simulink model "RoboticFish_NGC"  (R2023b)
settings: Solver=ode4  StartTime=0.0  StopTime=89  FixedStep=0.00025  RelTol=1e-3  EnableMultiTasking=on
undefined symbols (not defined in the file): Ref, uCMD
libraries: sharedutil x11, slpidlib x8, dspsigops x2, matrix_library x1, SignalEditorBlockLib x1, vrlib x1
(part 3 of 3)

== system RoboticFish_NGC/VRML /Estimate States/Subsystem ==
  Position : Inport
  nu_B : Inport  Port=2
  Bus Creator : BusCreator  Inputs=6
  Bus Creator1 : BusCreator  Inputs=6
  Bus Creator2 : BusCreator  Inputs=2
  Selector : Selector  InputPortWidth=6  IndexOptions=Index vector (dialog)  Indices=[1]  OutputSizes=1
  Selector1 : Selector  InputPortWidth=6  IndexOptions=Index vector (dialog)  Indices=[2]  OutputSizes=1
  Selector10 : Selector  InputPortWidth=6  IndexOptions=Index vector (dialog)  Indices=[5]  OutputSizes=1
  Selector11 : Selector  InputPortWidth=6  IndexOptions=Index vector (dialog)  Indices=[6]  OutputSizes=1
  Selector2 : Selector  InputPortWidth=6  IndexOptions=Index vector (dialog)  Indices=[3]  OutputSizes=1
  Selector3 : Selector  InputPortWidth=6  IndexOptions=Index vector (dialog)  Indices=[4]  OutputSizes=1
  Selector4 : Selector  InputPortWidth=6  IndexOptions=Index vector (dialog)  Indices=[5]  OutputSizes=1
  Selector5 : Selector  InputPortWidth=6  IndexOptions=Index vector (dialog)  Indices=[6]  OutputSizes=1
  Selector6 : Selector  InputPortWidth=6  IndexOptions=Index vector (dialog)  Indices=[1]  OutputSizes=1
  Selector7 : Selector  InputPortWidth=6  IndexOptions=Index vector (dialog)  Indices=[2]  OutputSizes=1
  Selector8 : Selector  InputPortWidth=6  IndexOptions=Index vector (dialog)  Indices=[3]  OutputSizes=1
  Selector9 : Selector  InputPortWidth=6  IndexOptions=Index vector (dialog)  Indices=[4]  OutputSizes=1
  State Estimate : Outport  VectorParamsAs1DForOutWhenUnconnected=off
  wires:
  Position/1 -> Selector5/1, Selector4/1, Selector3/1, Selector2/1, Selector1/1, Selector/1
  Selector/1 -> Bus Creator/1  "X"
  Selector1/1 -> Bus Creator/2  "Y"
  Selector2/1 -> Bus Creator/3  "Z"
  Selector3/1 -> Bus Creator/4  "Roll"
  Selector4/1 -> Bus Creator/5  "Pitch"
  Selector5/1 -> Bus Creator/6  "Yaw"
  nu_B/1 -> Selector8/1, Selector7/1, Selector6/1, Selector11/1, Selector10/1, Selector9/1
  Selector6/1 -> Bus Creator1/1  "u"
  Selector7/1 -> Bus Creator1/2  "v"
  Selector8/1 -> Bus Creator1/3  "w"
  Selector9/1 -> Bus Creator1/4  "p"
  Selector10/1 -> Bus Creator1/5  "q"
  Selector11/1 -> Bus Creator1/6  "r"
  Bus Creator/1 -> Bus Creator2/1  "Position"
  Bus Creator1/1 -> Bus Creator2/2  "Velocity"
  Bus Creator2/1 -> State Estimate/1

== system RoboticFish_NGC/VRML /RF Position and Rotation to VR Translation and Rotation/Orientation to VR Rotation ==
  Orientation : Inport
  Add : Sum  Inputs=4
  Constant1 : Constant  Value=[0; 0; 0; 0]
  Demux : Demux
  Demux1 : Demux
  Gain : Gain  Gain=2
  Gain1 : Gain  Gain=-1
  Gain2 : Gain  Gain=-1
  Math Function : Math  Operator=square  SignedPower=on
  Math Function1 : Math  Operator=reciprocal  SignedPower=on
  Mux : Mux
  Product1 : Product
  Sqrt : Sqrt
  Switch : Switch  Criteria=u2 > Threshold  SaturateOnIntegerOverflow=off  InputSameDT=off
  Trigonometric Function : Trigonometry  Operator=acos
  VR Rotation : Outport  VectorParamsAs1DForOutWhenUnconnected=off
  wires:
  Add/1 -> Sqrt/1
  Demux/2 -> Add/2
  Constant1/1 -> Switch/3
  Demux/3 -> Add/3
  Orientation/1 -> Product1/1, Math Function/1
  Sqrt/1 -> Math Function1/1, Switch/2
  Math Function1/1 -> Product1/2
  Demux/4 -> Add/4
  Demux/1 -> Add/1
  Math Function/1 -> Demux/1
  Product1/1 -> Switch/1
  Trigonometric Function/1 -> Gain/1
  Gain/1 -> Mux/4
  Mux/1 -> VR Rotation/1
  Switch/1 -> Demux1/1
  Demux1/1 -> Trigonometric Function/1  "q0"
  Demux1/2 -> Gain1/1  "q1"
  Demux1/3 -> Mux/1  "q2"
  Demux1/4 -> Gain2/1  "q3"
  Gain2/1 -> Mux/2
  Gain1/1 -> Mux/3

== system RoboticFish_NGC/VRML /RF Position and Rotation to VR Translation and Rotation/Position to VR Translation ==
  Position : Inport
  Demux : Demux  Outputs=3
  Gain : Gain  Gain=-1
  Gain1 : Gain  Gain=-1
  Mux : Mux  Inputs=3
  VR Translation : Outport  VectorParamsAs1DForOutWhenUnconnected=off
  wires:
  Position/1 -> Demux/1
  Demux/1 -> Gain/1  "x"
  Demux/2 -> Mux/1  "y"
  Demux/3 -> Gain1/1  "z"
  Mux/1 -> VR Translation/1
  Gain1/1 -> Mux/2
  Gain/1 -> Mux/3

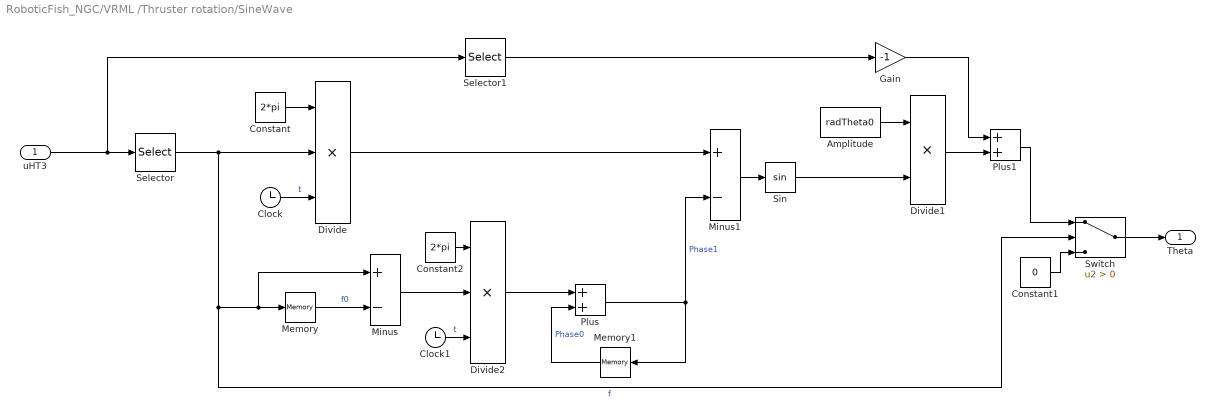
== system RoboticFish_NGC/VRML /Thruster rotation/SineWave ==
  uHT3 : Inport
  Amplitude : Constant  Value=radTheta0
  Clock : Clock
  Clock1 : Clock
  Constant : Constant  Value=2*pi
  Constant1 : Constant  Value=0
  Constant2 : Constant  Value=2*pi
  Divide : Product  Inputs=***
  Divide1 : Product  Inputs=**
  Divide2 : Product  Inputs=***
  Gain : Gain  Gain=-1
  Memory : Memory
  Memory1 : Memory
  Minus : Sum  Inputs=+-
  Minus1 : Sum  Inputs=+-
  Plus : Sum
  Plus1 : Sum
  Selector : Selector  InputPortWidth=2  IndexOptions=Index vector (dialog)  Indices=[1]  OutputSizes=1
  Selector1 : Selector  InputPortWidth=2  IndexOptions=Index vector (dialog)  Indices=[2]  OutputSizes=1
  Sin : Trigonometry
  Switch : Switch  Criteria=u2 > Threshold  SaturateOnIntegerOverflow=off  InputSameDT=off
  Theta : Outport  VectorParamsAs1DForOutWhenUnconnected=off
  wires:
  Constant/1 -> Divide/1
  uHT3/1 -> Selector1/1, Selector/1
  Clock/1 -> Divide/3  "t"
  Amplitude/1 -> Divide1/1
  Memory/1 -> Minus/2  "f0"
  Memory1/1 -> Plus/2  "Phase0"
  Plus/1 -> Memory1/1, Minus1/2  "Phase1"
  Divide/1 -> Minus1/1
  Minus/1 -> Divide2/2
  Divide2/1 -> Plus/1
  Minus1/1 -> Sin/1
  Sin/1 -> Divide1/2
  Selector/1 -> Switch/2, Minus/1, Memory/1, Divide/2  "f"
  Divide1/1 -> Plus1/2
  Selector1/1 -> Gain/1
  Plus1/1 -> Switch/1
  Gain/1 -> Plus1/1
  Constant1/1 -> Switch/3
  Switch/1 -> Theta/1
  Clock1/1 -> Divide2/3  "t"
  Constant2/1 -> Divide2/1

== system RoboticFish_NGC/VRML /WayPoint Position and Rotation To VR Translation and Rotation/Way point Position to VR Translation ==
  Position : Inport
  Demux : Demux  Outputs=3
  Gain : Gain  Gain=-1
  Gain1 : Gain  Gain=-1
  Mux : Mux  Inputs=3
  VR Translation : Outport  VectorParamsAs1DForOutWhenUnconnected=off
  wires:
  Gain/1 -> Mux/3
  Gain1/1 -> Mux/2
  Mux/1 -> VR Translation/1
  Demux/3 -> Gain1/1  "z"
  Demux/2 -> Mux/1  "y"
  Demux/1 -> Gain/1  "x"
  Position/1 -> Demux/1

== system RoboticFish_NGC/Guidance and Control system/ Control system/Control Allocator/Pseudoinverse choice ==
  note: Control Allocation choice
      |
      | The different matrix are used to select different actuators
      | The matrix is T which is the force coefficients pseudoinverse
      | matrix.
      | Matrix 1 - Only lateral propeller for horizontal plane
      | & pectoral fin for depth
      | Matrix 2 - surge motion by means of the caudal fin (HT3) & the
      | lateral propellers for steering & the pectoral fins are used
      | for the depth
      | Matrix 3 -surge force control, 𝜏𝑋, is null. All propellers are
      | switched off.
      | it could happen that the 𝑧 coordinate of the reference has not yet
      | been reached, in which case the control system automatically
      | activates the vertical propeller (VT1) to reach the target
      | Matrix 4 -> utilizza propulsori laterali
      | 𝑇4 + is used both in the case of “Only Propellers” and in the case of “Normal”. In this way the lateral propellers are used as brake. Note that the surge motion control and depth control are treated separately, therefore the force coefficient for the vertical propeller VT1 remains unchanged
      | Matrix 5 -> Only caudal fin
      | Si ha solo la spinta della coda per 𝜏𝑋, non viene compensato nè 𝜏N nè 𝜏Z. Per frenare verrà tolta alimentazione motore e si arriverà al punto desiderato per inerzia.
  Tin : Inport
  Actuators Choice : Inport  Port=2
  Matrix 1 : Constant  Value="[ 0 0 0 ;  0 0 0 ; 0.1 1  0;  0.1 -1  0;  0 0 1 ; 0 0 1  ;0  0 0]"
  Matrix 2 : Constant  Value="[ 1 0 0 ; 0 0 0 ;0 1 0 ;  0 -1 0 ;  0 0 1 ;  0 0 1 ; 0 0 0 ]"
  Matrix 3 : Constant  Value="[ 0 0 0 ;0  0 0; 0 0 0;  0 0 0;  0 0 0; 0 0 0;0 0 1]"
  Matrix 4 : Constant  Value="[ 0 0 0;0 0 0 ; -1 0 0 ;  -1 0 0 ;  0 0  0; 0 0 0;0 0 1]"
  Matrix 5 : Constant  Value="[ 1 0 0; 0 1 0; 0 0 0;  0 0 0;  0 0 0; 0 0 0;0 0 0]"
  Selector : Selector  InputPortWidth=3  IndexOptions=Index vector (dialog)  Indices=[1]  OutputSizes=1
  Switch : Switch  Criteria=u2 > Threshold  SaturateOnIntegerOverflow=off  InputSameDT=off
  Switch1 : Switch  Criteria=u2 > Threshold  Threshold=0.2  SaturateOnIntegerOverflow=off  InputSameDT=off
  Switch2 : Switch  Criteria=u2 > Threshold  Threshold=0.05  SaturateOnIntegerOverflow=off  InputSameDT=off
  Switch3 : Switch  Criteria=u2 > Threshold  Threshold=1  SaturateOnIntegerOverflow=off  InputSameDT=off
  Pseudoinverse : Outport  VectorParamsAs1DForOutWhenUnconnected=off
  wires:
  Tin/1 -> Selector/1
  Matrix 1/1 -> Switch/1
  Actuators Choice/1 -> Switch/2, Switch3/2
  Switch/1 -> Switch1/1
  Switch1/1 -> Switch2/1
  Selector/1 -> Switch2/2, Switch1/2
  Matrix 2/1 -> Switch/3
  Matrix 3/1 -> Switch1/3
  Matrix 4/1 -> Switch2/3
  Switch2/1 -> Switch3/3
  Switch3/1 -> Pseudoinverse/1
  Matrix 5/1 -> Switch3/1

== system RoboticFish_NGC/Guidance and Control system/ Control system/Control Allocator/Saturation limits ==
  InBus : Inport
  Bus Creator : BusCreator  Inputs=7
  Saturation Thetastr_HT3 : Saturate  UpperLimit=1.3090  LowerLimit=-1.3090
  Saturation f_HT3 : Saturate  UpperLimit=4  LowerLimit=0
  Saturation uHT1 : Saturate  UpperLimit=1  LowerLimit=-1
  Saturation uHT2 : Saturate  UpperLimit=1  LowerLimit=-1
  Saturation uVT1 : Saturate  UpperLimit=1  LowerLimit=-1
  Saturation uVT2 : Saturate  UpperLimit=1  LowerLimit=-1
  Saturation uVT3 : Saturate  UpperLimit=1  LowerLimit=-1
  Selector Thetastr_HT3 : Selector  InputPortWidth=7  IndexOptions=Index vector (dialog)  Indices=[2]  OutputSizes=1
  Selector f_HT3 : Selector  InputPortWidth=7  IndexOptions=Index vector (dialog)  Indices=[1]  OutputSizes=1
  Selector uHT1 : Selector  InputPortWidth=7  IndexOptions=Index vector (dialog)  Indices=[3]  OutputSizes=1
  Selector uHT2 : Selector  InputPortWidth=7  IndexOptions=Index vector (dialog)  Indices=[4]  OutputSizes=1
  Selector uVT1 : Selector  InputPortWidth=7  IndexOptions=Index vector (dialog)  Indices=[7]  OutputSizes=1
  Selector uVT3 : Selector  InputPortWidth=7  IndexOptions=Index vector (dialog)  Indices=[6]  OutputSizes=1
  Selector5 uVT2 : Selector  InputPortWidth=7  IndexOptions=Index vector (dialog)  Indices=[5]  OutputSizes=1
  uCMD : Outport  VectorParamsAs1DForOutWhenUnconnected=off
  wires:
  Saturation uVT3/1 -> Bus Creator/7  "uVT3"
  Saturation uVT2/1 -> Bus Creator/6  "uVT2"
  Saturation uVT1/1 -> Bus Creator/5  "uVT1"
  Saturation uHT2/1 -> Bus Creator/4  "uHT2"
  Selector uHT1/1 -> Saturation uHT1/1
  Saturation uHT1/1 -> Bus Creator/3  "uHT1"
  Selector Thetastr_HT3/1 -> Saturation Thetastr_HT3/1
  Saturation f_HT3/1 -> Bus Creator/1  "f_HT3"
  Bus Creator/1 -> uCMD/1
  Selector uVT3/1 -> Saturation uVT3/1
  Selector5 uVT2/1 -> Saturation uVT2/1
  Selector uVT1/1 -> Saturation uVT1/1
  Selector uHT2/1 -> Saturation uHT2/1
  InBus/1 -> Selector f_HT3/1, Selector Thetastr_HT3/1, Selector uHT1/1, Selector uHT2/1, Selector5 uVT2/1, Selector uVT3/1, Selector uVT1/1
  Saturation Thetastr_HT3/1 -> Bus Creator/2  "Thetastr_HT3"
  Selector f_HT3/1 -> Saturation f_HT3/1

== system RoboticFish_NGC/Guidance and Control system/ Control system/Control Law/Switch Case Action Subsystem ==
  LOS : Inport
  Action Port : ActionPort  ActionPortLabel=case [ 0 ]:
  D : Outport
  wires:
  LOS/1 -> D/1

== system RoboticFish_NGC/Guidance and Control system/ Control system/Control Law/Switch Case Action Subsystem1 ==
  LOS : Inport
  Action Port : ActionPort  ActionPortLabel=case [ 1 ]:
  D : Outport
  wires:
  LOS/1 -> D/1

== system RoboticFish_NGC/Guidance and Control system/ Control system/Control Law/Switch Case Action Subsystem2 ==
  LOS : Inport
  Action Port : ActionPort  ActionPortLabel=case [ 2 ]:
  D : Outport
  wires:
  LOS/1 -> D/1

== system RoboticFish_NGC/Guidance and Control system/ Control system/Control Law/Switch Case Action Subsystem3 ==
  LOS : Inport
  Action Port : ActionPort  ActionPortLabel=case [ 0 ]:
  Ze : Outport
  wires:
  LOS/1 -> Ze/1

== system RoboticFish_NGC/Guidance and Control system/ Control system/Control Law/Switch Case Action Subsystem4 ==
  LOS : Inport
  Action Port : ActionPort  ActionPortLabel=case [ 1 ]:
  Ze : Outport
  wires:
  LOS/1 -> Ze/1

== system RoboticFish_NGC/Guidance and Control system/ Control system/Control Law/Switch Case Action Subsystem5 ==
  LOS : Inport
  Action Port : ActionPort  ActionPortLabel=case [ 2 ]:
  D : Outport
  wires:
  LOS/1 -> D/1

== system RoboticFish_NGC/Guidance and Control system/ Control system/Control Law/Switch Case Action Subsystem6 ==
  LOS : Inport
  Action Port : ActionPort  ActionPortLabel=case [ 0 1 ]:
  D : Outport
  wires:
  LOS/1 -> D/1

== system RoboticFish_NGC/Guidance and Control system/ Control system/Control Law/Switch Case Action Subsystem7 ==
  LOS : Inport
  Action Port : ActionPort  ActionPortLabel=case [ 2 ]:
  D : Outport
  wires:
  LOS/1 -> D/1

== system RoboticFish_NGC/Guidance and Control system/ Control system/Control Law/Unwrap ==
  yaw in : Inport
  Gain : Gain  Gain=pi/180
  Gain1 : Gain  Gain=180/pi
  Unwrap : dspsigops/Unwrap  tol=pi  InputProcessing=Columns as channels (frame based)  running=off
  yaw out : Outport  VectorParamsAs1DForOutWhenUnconnected=off
  wires:
  Gain1/1 -> yaw out/1
  Unwrap/1 -> Gain1/1
  Gain/1 -> Unwrap/1
  yaw in/1 -> Gain/1

== system RoboticFish_NGC/Robotic-Fish Model & PropulsionSystem/Propulsion System/Horizontal Force and Moment (Tau_H)/Tau_HT3 (Tau_Caudal_Fin) ==
  "[U uHT3 t]" : Inport
  Bus Creator : BusCreator  Inputs=6
  Calculation_Tau_HT3 : Subsystem
  Constant3 : Constant  Value=[0;0;0;0;0;0]
  Fsurge : Fcn  Expr=Kt1*u(2)*u(2)*(Kt0+Kt2*sin(4*pi*u(3)*u(2)+beta))
  Fsway : Fcn  Expr=Kl1*u(2)*u(2)*Kl2*cos(2*pi*u(3)*u(2)+sigma)
  Myaw : Fcn  Expr=Km1*u(2)*u(2)*Km2*cos(2*pi*u(3)*u(2)+epsilon)
  Selector : Selector  InputPortWidth=4  IndexOptions=Index vector (dialog)  Indices=[ 3]  OutputSizes=1
  Selector1 : Selector  InputPortWidth=4  IndexOptions=Index vector (dialog)  Indices=[1 2 4]  OutputSizes=1
  Selector3 : Selector  InputPortWidth=3  IndexOptions=Index vector (dialog)  Indices=[2]  OutputSizes=1
  SinCos : Trigonometry  Operator=sincos
  Switch : Switch  Criteria=u2 > Threshold  SaturateOnIntegerOverflow=off  InputSameDT=off
  Tau_HT3 : Outport  VectorParamsAs1DForOutWhenUnconnected=off
  wires:
  Calculation_Tau_HT3/1(Tau_HT3) -> Switch/1  "[Tau_surge_HT3 Tau_sway_HT3 0 0 0 Tau_yaw_HT3]"
  Switch/1 -> Tau_HT3/1
  Constant3/1 -> Switch/3
  "[U uHT3 t]"/1 -> Selector/1, Selector1/1
  Selector3/1 -> Switch/2  "f"
  Selector1/1 -> Fsurge/1, Selector3/1, Bus Creator/6, Myaw/1, Fsway/1  "[U f_HT3 t]"
  SinCos/1 -> Bus Creator/1  "sin(Thetastr_HT3)"
  SinCos/2 -> Bus Creator/2  "cos(Thetastr_HT3)"
  Fsurge/1 -> Bus Creator/3  "Fsurge"
  Fsway/1 -> Bus Creator/4  "Fsway"
  Myaw/1 -> Bus Creator/5  "Myaw"
  Bus Creator/1 -> Calculation_Tau_HT3/1(InBus)
  Selector/1 -> SinCos/1

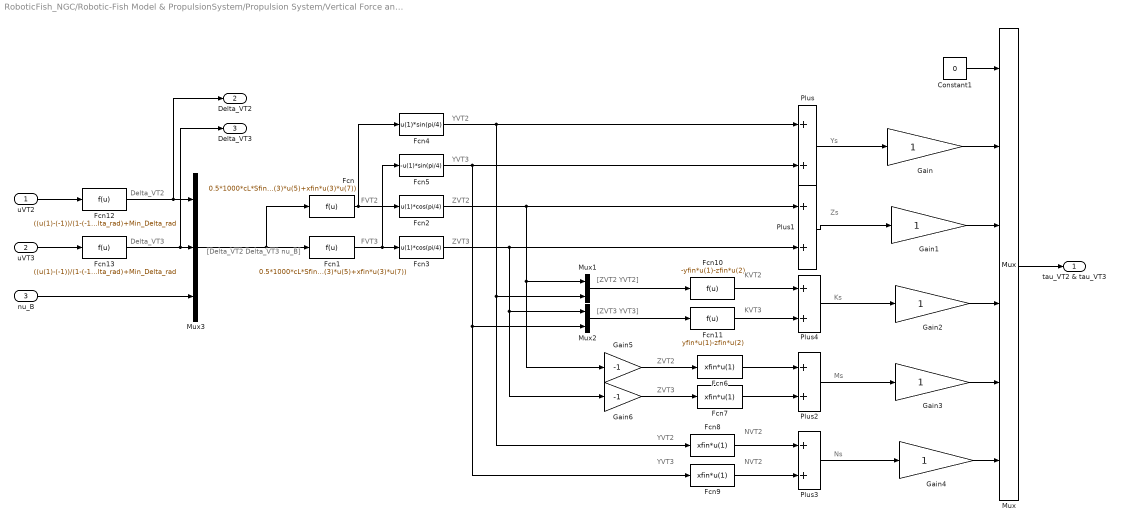
== system RoboticFish_NGC/Robotic-Fish Model & PropulsionSystem/Propulsion System/Vertical Force and Moment (Tau_V)/Tau_VT2&VT3 (Pectoral Fin) ==
  note: Ys
  note: [Delta_VT2 Delta_VT3 nu_B]
  note: Delta_VT2
  note: [ZVT2 YVT2]
  note: FVT2
  note: FVT3
  note: ZVT2
  note: ZVT3
  note: YVT2
  note: YVT3
  note: [ZVT3 YVT3]
  note: KVT3
  note: KVT2
  note: NVT2
  note: NVT2
  note: ZVT3
  note: ZVT2
  note: YVT2
  note: YVT3
  note: Delta_VT3
  note: Zs
  note: Ks
  note: Ms
  note: Ns
  "uVT2 " : Inport
  uVT3 : Inport  Port=2
  nu_B : Inport  Port=3
  Constant1 : Constant  Value=0
  Fcn : Fcn  Expr=0.5*1000*cL*Sfin*(u(3)^2*u(1)+u(3)*u(5)+xfin*u(3)*u(7))
  Fcn1 : Fcn  Expr=0.5*1000*cL*Sfin*(u(3)^2*u(2)+u(3)*u(5)+xfin*u(3)*u(7))
  Fcn10 : Fcn  Expr=-yfin*u(1)-zfin*u(2)
  Fcn11 : Fcn  Expr=yfin*u(1)-zfin*u(2)
  Fcn12 : Fcn  Expr=((u(1)-(-1))/(1-(-1)))*(Max_Delta_rad-Min_Delta_rad)+Min_Delta_rad
  Fcn13 : Fcn  Expr=((u(1)-(-1))/(1-(-1)))*(Max_Delta_rad-Min_Delta_rad)+Min_Delta_rad
  Fcn2 : Fcn  Expr=u(1)*cos(pi/4)
  Fcn3 : Fcn  Expr=u(1)*cos(pi/4)
  Fcn4 : Fcn  Expr=u(1)*sin(pi/4)
  Fcn5 : Fcn  Expr=-u(1)*sin(pi/4)
  Fcn{6..9} (4 alike) : Fcn  Expr=xfin*u(1)
  Gain{,1..4} (5 alike) : Gain
  Gain5 : Gain  Gain=-1
  Gain6 : Gain  Gain=-1
  Mux : Mux  Inputs=6
  Mux1 : Mux  Inputs=2
  Mux2 : Mux  Inputs=2
  Mux3 : Mux  Inputs=3
  Plus{,1..4} (5 alike) : Sum
  "tau_VT2 & tau_VT3 " : Outport  VectorParamsAs1DForOutWhenUnconnected=off
  Delta_VT2 : Outport  Port=2  VectorParamsAs1DForOutWhenUnconnected=off
  Delta_VT3 : Outport  Port=3  VectorParamsAs1DForOutWhenUnconnected=off
  wires:
  Constant1/1 -> Mux/1
  Mux/1 -> "tau_VT2 & tau_VT3 "/1
  Fcn/1 -> Fcn4/1, Fcn2/1
  Fcn1/1 -> Fcn5/1, Fcn3/1
  Fcn4/1 -> Plus/1, Fcn8/1, Mux1/2
  Fcn5/1 -> Fcn9/1, Mux2/2, Plus/2
  Fcn2/1 -> Gain5/1, Mux1/1, Plus1/1
  Fcn3/1 -> Plus1/2, Gain6/1, Mux2/1
  Mux1/1 -> Fcn10/1
  Mux2/1 -> Fcn11/1
  Fcn10/1 -> Plus4/1
  Fcn11/1 -> Plus4/2
  Fcn9/1 -> Plus3/2
  Fcn8/1 -> Plus3/1
  Gain6/1 -> Fcn7/1
  Gain5/1 -> Fcn6/1
  Plus/1 -> Gain/1
  Plus4/1 -> Gain2/1
  Plus3/1 -> Gain4/1
  "uVT2 "/1 -> Fcn12/1
  uVT3/1 -> Fcn13/1
  Fcn12/1 -> Delta_VT2/1, Mux3/1
  Fcn13/1 -> Delta_VT3/1, Mux3/2
  nu_B/1 -> Mux3/3
  Mux3/1 -> Fcn/1, Fcn1/1
  Gain/1 -> Mux/2
  Gain2/1 -> Mux/4
  Gain4/1 -> Mux/6
  Plus1/1 -> Gain1/1
  Gain1/1 -> Mux/3
  Plus2/1 -> Gain3/1
  Fcn6/1 -> Plus2/1
  Fcn7/1 -> Plus2/2
  Gain3/1 -> Mux/5

== system RoboticFish_NGC/Robotic-Fish Model & PropulsionSystem/RF Dynamics and Kinematics (Attitude rappresentation: Quaternions)/6 DOF transformation/E1(e) ==
  note: q1,q2,q3
  note: qo
  e : Inport
  Gain : Gain  Gain=2  SaturateOnIntegerOverflow=on  OutDataTypeStr=Inherit: Same as input  ParamDataTypeStr=Inherit: Same as input
  "Gain " : Gain  Gain=2  SaturateOnIntegerOverflow=on  OutDataTypeStr=Inherit: Same as input  ParamDataTypeStr=Inherit: Same as input
  I (3x3) : Constant  Value=eye(3)
  Matrix Multiply : Product  Multiplication=Matrix(*)
  Product : Product  SaturateOnIntegerOverflow=on  OutDataTypeStr=Inherit: Same as first input
  Selector : Selector  InputPortWidth=4  IndexOptions=Index vector (dialog)  Indices=[1]  OutputSizes=1
  Selector1 : Selector  InputPortWidth=4  IndexOptions=Index vector (dialog)  Indices=[2 3 4]  OutputSizes=1
  Skew Symmetrical Operator : Subsystem
  Sum : Sum  Inputs=+++  SaturateOnIntegerOverflow=on
  E1 : Outport  VectorParamsAs1DForOutWhenUnconnected=off
  wires:
  e/1 -> Selector/1, Selector1/1
  Selector/1 -> "Gain "/1  "eta"
  Selector1/1 -> Skew Symmetrical Operator/1(v)  "eps"
  Skew Symmetrical Operator/1(S(V)) -> Matrix Multiply/1, Matrix Multiply/2, Product/2
  Matrix Multiply/1 -> Gain/1
  "Gain "/1 -> Product/1
  I (3x3)/1 -> Sum/1
  Product/1 -> Sum/2
  Gain/1 -> Sum/3
  Sum/1 -> E1/1

== system RoboticFish_NGC/Robotic-Fish Model & PropulsionSystem/RF Dynamics and Kinematics (Attitude rappresentation: Quaternions)/6 DOF transformation/E2(e) ==
  note: q=(q1,q2,q3)
  note: q0
  e : Inport
  Gain : Gain  Gain=0.5  SaturateOnIntegerOverflow=on  OutDataTypeStr=Inherit: Same as input  ParamDataTypeStr=Inherit: Same as input
  Gain1 : Gain  Gain=-1  SaturateOnIntegerOverflow=on  OutDataTypeStr=Inherit: Same as input  ParamDataTypeStr=Inherit: Same as input
  I (3x3) : Constant  Value=eye(3)
  Matrix Concatenation : Concatenate  Mode=Multidimensional array
  Product : Product  SaturateOnIntegerOverflow=on  OutDataTypeStr=Inherit: Same as first input
  Selector : Selector  InputPortWidth=4  IndexOptions=Index vector (dialog)  Indices=[1]  OutputSizes=1
  Selector1 : Selector  InputPortWidth=4  IndexOptions=Index vector (dialog)  Indices=[2 3 4]  OutputSizes=1
  Skew Symmetrical Operator : Subsystem
  Sum : Sum  SaturateOnIntegerOverflow=on
  Transpose : Math  Operator=transpose  SignedPower=on
  E2 : Outport  VectorParamsAs1DForOutWhenUnconnected=off
  wires:
  Selector1/1 -> Skew Symmetrical Operator/1(v), Transpose/1  "eps"
  Selector/1 -> Product/2  "eta"
  e/1 -> Selector1/1, Selector/1
  I (3x3)/1 -> Product/1
  Product/1 -> Sum/1  "eta*I"
  Skew Symmetrical Operator/1(S(V)) -> Sum/2  "S(eps)"
  Transpose/1 -> Gain1/1
  Gain1/1 -> Matrix Concatenation/1  "-eps^T"
  Sum/1 -> Matrix Concatenation/2
  Matrix Concatenation/1 -> Gain/1
  Gain/1 -> E2/1

== system RoboticFish_NGC/Robotic-Fish Model & PropulsionSystem/RF Dynamics and Kinematics (Attitude rappresentation: Quaternions)/Added Mass Coriolis and centripetal matrix/Skew Symmetrical Operator ==
  v : Inport
  Constant : Constant  Value=0
  Create 3x3 Matrix : sharedutil/Create 3x3 Matrix  aMode=aMode
  Demux : Demux  Outputs=3
      settings: DisplayOption=none
  Gain : Gain  Gain=-1  SaturateOnIntegerOverflow=on  OutDataTypeStr=Inherit: Same as input  ParamDataTypeStr=Inherit: Same as input
  Gain1 : Gain  Gain=-1  SaturateOnIntegerOverflow=on  OutDataTypeStr=Inherit: Same as input  ParamDataTypeStr=Inherit: Same as input
  Gain2 : Gain  Gain=-1  SaturateOnIntegerOverflow=on  OutDataTypeStr=Inherit: Same as input  ParamDataTypeStr=Inherit: Same as input
  S(V) : Outport  VectorParamsAs1DForOutWhenUnconnected=off
  wires:
  v/1 -> Demux/1
  Create 3x3 Matrix/1 -> S(V)/1
  Gain2/1 -> Create 3x3 Matrix/2  "-v(3)"
  Gain1/1 -> Create 3x3 Matrix/7  "-v(2)"
  Gain/1 -> Create 3x3 Matrix/6  "-v(1)"
  Demux/3 -> Create 3x3 Matrix/4, Gain2/1  "v(3)"
  Demux/2 -> Create 3x3 Matrix/3, Gain1/1  "v(2)"
  Demux/1 -> Create 3x3 Matrix/8, Gain/1  "v(1)"
  Constant/1 -> Create 3x3 Matrix/5, Create 3x3 Matrix/9, Create 3x3 Matrix/1

== system RoboticFish_NGC/Robotic-Fish Model & PropulsionSystem/RF Dynamics and Kinematics (Attitude rappresentation: Quaternions)/Added Mass Coriolis and centripetal matrix/Skew Symmetrical Operator  ==
  v : Inport
  Constant : Constant  Value=0
  Create 3x3 Matrix : sharedutil/Create 3x3 Matrix  aMode=aMode
  Demux : Demux  Outputs=3
      settings: DisplayOption=none
  Gain : Gain  Gain=-1  SaturateOnIntegerOverflow=on  OutDataTypeStr=Inherit: Same as input  ParamDataTypeStr=Inherit: Same as input
  Gain1 : Gain  Gain=-1  SaturateOnIntegerOverflow=on  OutDataTypeStr=Inherit: Same as input  ParamDataTypeStr=Inherit: Same as input
  Gain2 : Gain  Gain=-1  SaturateOnIntegerOverflow=on  OutDataTypeStr=Inherit: Same as input  ParamDataTypeStr=Inherit: Same as input
  S(V) : Outport  VectorParamsAs1DForOutWhenUnconnected=off
  wires:
  Constant/1 -> Create 3x3 Matrix/1, Create 3x3 Matrix/9, Create 3x3 Matrix/5
  Demux/1 -> Gain/1, Create 3x3 Matrix/8  "v(1)"
  Demux/2 -> Gain1/1, Create 3x3 Matrix/3  "v(2)"
  Demux/3 -> Gain2/1, Create 3x3 Matrix/4  "v(3)"
  Gain/1 -> Create 3x3 Matrix/6  "-v(1)"
  Gain1/1 -> Create 3x3 Matrix/7  "-v(2)"
  Gain2/1 -> Create 3x3 Matrix/2  "-v(3)"
  Create 3x3 Matrix/1 -> S(V)/1
  v/1 -> Demux/1

== system RoboticFish_NGC/Robotic-Fish Model & PropulsionSystem/RF Dynamics and Kinematics (Attitude rappresentation: Quaternions)/Quaternion normalisation/norm 1x4 vector ==
  Inport : Inport
  Plus : Sum  Inputs=++++
  Selector : Selector  InputPortWidth=4  IndexOptions=Index vector (dialog)  Indices=[1]  OutputSizes=1
  Selector1 : Selector  InputPortWidth=4  IndexOptions=Index vector (dialog)  Indices=[2]  OutputSizes=1
  Selector2 : Selector  InputPortWidth=4  IndexOptions=Index vector (dialog)  Indices=[3]  OutputSizes=1
  Selector3 : Selector  InputPortWidth=4  IndexOptions=Index vector (dialog)  Indices=[4]  OutputSizes=1
  Sqrt : Sqrt
  Square{,1..3} (4 alike) : Math  Operator=square  SignedPower=on
  norm : Outport  VectorParamsAs1DForOutWhenUnconnected=off
  wires:
  Square2/1 -> Plus/3
  Square1/1 -> Plus/2
  Square/1 -> Plus/1
  Inport/1 -> Selector3/1, Selector2/1, Selector/1, Selector1/1
  Square3/1 -> Plus/4
  Selector3/1 -> Square3/1
  Plus/1 -> Sqrt/1
  Selector2/1 -> Square2/1
  Sqrt/1 -> norm/1
  Selector1/1 -> Square1/1
  Selector/1 -> Square/1

== system RoboticFish_NGC/Robotic-Fish Model & PropulsionSystem/RF Dynamics and Kinematics (Attitude rappresentation: Quaternions)/Restoring forces/E1(e) ==
  e : Inport
  Gain : Gain  Gain=2  SaturateOnIntegerOverflow=on  OutDataTypeStr=Inherit: Same as input  ParamDataTypeStr=Inherit: Same as input
  "Gain " : Gain  Gain=2  SaturateOnIntegerOverflow=on  OutDataTypeStr=Inherit: Same as input  ParamDataTypeStr=Inherit: Same as input
  I (3x3) : Constant  Value=eye(3)
  Matrix Multiply : Product  Multiplication=Matrix(*)
  Product : Product  SaturateOnIntegerOverflow=on  OutDataTypeStr=Inherit: Same as first input
  Selector : Selector  InputPortWidth=4  IndexOptions=Index vector (dialog)  Indices=[1]  OutputSizes=1
  Selector1 : Selector  InputPortWidth=4  IndexOptions=Index vector (dialog)  Indices=[2 3 4]  OutputSizes=1
  Skew Symmetrical Operator : Subsystem
  Sum : Sum  Inputs=+++  SaturateOnIntegerOverflow=on
  E1 : Outport  VectorParamsAs1DForOutWhenUnconnected=off
  wires:
  Sum/1 -> E1/1
  Gain/1 -> Sum/3
  Product/1 -> Sum/2
  I (3x3)/1 -> Sum/1
  "Gain "/1 -> Product/1
  Matrix Multiply/1 -> Gain/1
  Skew Symmetrical Operator/1(S(V)) -> Product/2, Matrix Multiply/2, Matrix Multiply/1
  Selector1/1 -> Skew Symmetrical Operator/1(v)  "eps"
  Selector/1 -> "Gain "/1  "eta"
  e/1 -> Selector1/1, Selector/1

== system RoboticFish_NGC/Robotic-Fish Model & PropulsionSystem/RF Dynamics and Kinematics (Attitude rappresentation: Quaternions)/Rigid-body Coriolis and centripetal matrix/Skew Symmetrical Operator  ==
  v : Inport
  Constant : Constant  Value=0
  Create 3x3 Matrix : sharedutil/Create 3x3 Matrix  aMode=aMode
  Demux : Demux  Outputs=3
      settings: DisplayOption=none
  Gain : Gain  Gain=-1  SaturateOnIntegerOverflow=on  OutDataTypeStr=Inherit: Same as input  ParamDataTypeStr=Inherit: Same as input
  Gain1 : Gain  Gain=-1  SaturateOnIntegerOverflow=on  OutDataTypeStr=Inherit: Same as input  ParamDataTypeStr=Inherit: Same as input
  Gain2 : Gain  Gain=-1  SaturateOnIntegerOverflow=on  OutDataTypeStr=Inherit: Same as input  ParamDataTypeStr=Inherit: Same as input
  S(V) : Outport  VectorParamsAs1DForOutWhenUnconnected=off
  wires:
  Constant/1 -> Create 3x3 Matrix/1, Create 3x3 Matrix/9, Create 3x3 Matrix/5
  Demux/1 -> Gain/1, Create 3x3 Matrix/8  "v(1)"
  Demux/2 -> Gain1/1, Create 3x3 Matrix/3  "v(2)"
  Demux/3 -> Gain2/1, Create 3x3 Matrix/4  "v(3)"
  Gain/1 -> Create 3x3 Matrix/6  "-v(1)"
  Gain1/1 -> Create 3x3 Matrix/7  "-v(2)"
  Gain2/1 -> Create 3x3 Matrix/2  "-v(3)"
  Create 3x3 Matrix/1 -> S(V)/1
  v/1 -> Demux/1

== system RoboticFish_NGC/Robotic-Fish Model & PropulsionSystem/RF Dynamics and Kinematics (Attitude rappresentation: Quaternions)/Rigid-body Coriolis and centripetal matrix/Skew Symmetrical Operator ==
  v : Inport
  Constant : Constant  Value=0
  Create 3x3 Matrix : sharedutil/Create 3x3 Matrix  aMode=aMode
  Demux : Demux  Outputs=3
      settings: DisplayOption=none
  Gain : Gain  Gain=-1  SaturateOnIntegerOverflow=on  OutDataTypeStr=Inherit: Same as input  ParamDataTypeStr=Inherit: Same as input
  Gain1 : Gain  Gain=-1  SaturateOnIntegerOverflow=on  OutDataTypeStr=Inherit: Same as input  ParamDataTypeStr=Inherit: Same as input
  Gain2 : Gain  Gain=-1  SaturateOnIntegerOverflow=on  OutDataTypeStr=Inherit: Same as input  ParamDataTypeStr=Inherit: Same as input
  S(V) : Outport  VectorParamsAs1DForOutWhenUnconnected=off
  wires:
  Constant/1 -> Create 3x3 Matrix/1, Create 3x3 Matrix/9, Create 3x3 Matrix/5
  Demux/1 -> Gain/1, Create 3x3 Matrix/8  "v(1)"
  Demux/2 -> Gain1/1, Create 3x3 Matrix/3  "v(2)"
  Demux/3 -> Gain2/1, Create 3x3 Matrix/4  "v(3)"
  Gain/1 -> Create 3x3 Matrix/6  "-v(1)"
  Gain1/1 -> Create 3x3 Matrix/7  "-v(2)"
  Gain2/1 -> Create 3x3 Matrix/2  "-v(3)"
  Create 3x3 Matrix/1 -> S(V)/1
  v/1 -> Demux/1

== system RoboticFish_NGC/Robotic-Fish Model & PropulsionSystem/RF Dynamics and Kinematics (Attitude rappresentation: Quaternions)/Rigid-body Coriolis and centripetal matrix/Skew Symmetrical Operator  ==
  v : Inport
  Constant : Constant  Value=0
  Create 3x3 Matrix : sharedutil/Create 3x3 Matrix  aMode=aMode
  Demux : Demux  Outputs=3
      settings: DisplayOption=none
  Gain : Gain  Gain=-1  SaturateOnIntegerOverflow=on  OutDataTypeStr=Inherit: Same as input  ParamDataTypeStr=Inherit: Same as input
  Gain1 : Gain  Gain=-1  SaturateOnIntegerOverflow=on  OutDataTypeStr=Inherit: Same as input  ParamDataTypeStr=Inherit: Same as input
  Gain2 : Gain  Gain=-1  SaturateOnIntegerOverflow=on  OutDataTypeStr=Inherit: Same as input  ParamDataTypeStr=Inherit: Same as input
  S(V) : Outport  VectorParamsAs1DForOutWhenUnconnected=off
  wires:
  v/1 -> Demux/1
  Create 3x3 Matrix/1 -> S(V)/1
  Gain2/1 -> Create 3x3 Matrix/2  "-v(3)"
  Gain1/1 -> Create 3x3 Matrix/7  "-v(2)"
  Gain/1 -> Create 3x3 Matrix/6  "-v(1)"
  Demux/3 -> Create 3x3 Matrix/4, Gain2/1  "v(3)"
  Demux/2 -> Create 3x3 Matrix/3, Gain1/1  "v(2)"
  Demux/1 -> Create 3x3 Matrix/8, Gain/1  "v(1)"
  Constant/1 -> Create 3x3 Matrix/5, Create 3x3 Matrix/9, Create 3x3 Matrix/1

== system RoboticFish_NGC/Robotic-Fish Model & PropulsionSystem/RF Dynamics and Kinematics (Attitude rappresentation: Quaternions)/Rigid-body Coriolis and centripetal matrix/Skew Symmetrical Operator   ==
  v : Inport
  Constant : Constant  Value=0
  Create 3x3 Matrix : sharedutil/Create 3x3 Matrix  aMode=aMode
  Demux : Demux  Outputs=3
      settings: DisplayOption=none
  Gain : Gain  Gain=-1  SaturateOnIntegerOverflow=on  OutDataTypeStr=Inherit: Same as input  ParamDataTypeStr=Inherit: Same as input
  Gain1 : Gain  Gain=-1  SaturateOnIntegerOverflow=on  OutDataTypeStr=Inherit: Same as input  ParamDataTypeStr=Inherit: Same as input
  Gain2 : Gain  Gain=-1  SaturateOnIntegerOverflow=on  OutDataTypeStr=Inherit: Same as input  ParamDataTypeStr=Inherit: Same as input
  S(V) : Outport  VectorParamsAs1DForOutWhenUnconnected=off
  wires:
  Constant/1 -> Create 3x3 Matrix/1, Create 3x3 Matrix/9, Create 3x3 Matrix/5
  Demux/1 -> Gain/1, Create 3x3 Matrix/8  "v(1)"
  Demux/2 -> Gain1/1, Create 3x3 Matrix/3  "v(2)"
  Demux/3 -> Gain2/1, Create 3x3 Matrix/4  "v(3)"
  Gain/1 -> Create 3x3 Matrix/6  "-v(1)"
  Gain1/1 -> Create 3x3 Matrix/7  "-v(2)"
  Gain2/1 -> Create 3x3 Matrix/2  "-v(3)"
  Create 3x3 Matrix/1 -> S(V)/1
  v/1 -> Demux/1

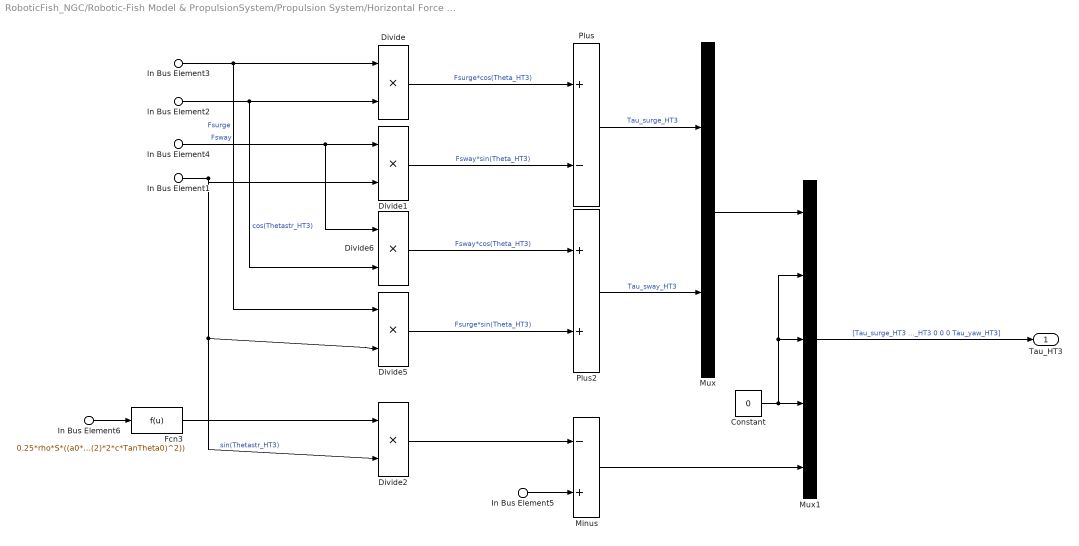
== system RoboticFish_NGC/Robotic-Fish Model & PropulsionSystem/Propulsion System/Horizontal Force and Moment (Tau_H)/Tau_HT3 (Tau_Caudal_Fin)/Calculation_Tau_HT3 ==
  In Bus Element1 : Inport  PortName=InBus  Element=sin(Thetastr_HT3)
  In Bus Element2 : Inport  PortName=InBus  Element=cos(Thetastr_HT3)
  In Bus Element3 : Inport  PortName=InBus  Element=Fsurge
  In Bus Element4 : Inport  PortName=InBus  Element=Fsway
  In Bus Element5 : Inport  PortName=InBus  Element=Myaw
  In Bus Element6 : Inport  PortName=InBus  Element=[U f_HT3 t]
  Constant : Constant  Value=0
  Divide{,1..2,5..6} (5 alike) : Product  Inputs=**
  Fcn3 : Fcn  Expr=0.25*rho*S*((a0*u(1)^2+a1*u(1)*u(2)*2*c*TanTheta0+a2*(u(2)*2*c*TanTheta0)^2))
  Minus : Sum  Inputs=-+
  Mux : Mux  Inputs=2
  Mux1 : Mux  Inputs=5
  Plus : Sum  Inputs=+-
  Plus2 : Sum
  Tau_HT3 : Outport  VectorParamsAs1DForOutWhenUnconnected=off
  wires:
  In Bus Element3/1 -> Divide5/1, Divide/1  "Fsurge"
  In Bus Element2/1 -> Divide/2, Divide6/2  "cos(Thetastr_HT3)"
  Divide/1 -> Plus/1  "Fsurge*cos(Theta_HT3)"
  Divide1/1 -> Plus/2  "Fsway*sin(Theta_HT3)"
  In Bus Element4/1 -> Divide1/1, Divide6/1  "Fsway"
  In Bus Element1/1 -> Divide1/2, Divide2/2, Divide5/2  "sin(Thetastr_HT3)"
  Divide6/1 -> Plus2/1  "Fsway*cos(Theta_HT3)"
  Divide5/1 -> Plus2/2  "Fsurge*sin(Theta_HT3)"
  In Bus Element6/1 -> Fcn3/1
  Fcn3/1 -> Divide2/1
  Divide2/1 -> Minus/1
  In Bus Element5/1 -> Minus/2
  Plus2/1 -> Mux/2  "Tau_sway_HT3"
  Plus/1 -> Mux/1  "Tau_surge_HT3"
  Mux/1 -> Mux1/1
  Minus/1 -> Mux1/5
  Constant/1 -> Mux1/2, Mux1/3, Mux1/4
  Mux1/1 -> Tau_HT3/1  "[Tau_surge_HT3 Tau_sway_HT3 0 0 0 Tau_yaw_HT3]"

== system RoboticFish_NGC/Robotic-Fish Model & PropulsionSystem/RF Dynamics and Kinematics (Attitude rappresentation: Quaternions)/6 DOF transformation/E1(e)/Skew Symmetrical Operator ==
  v : Inport
  Constant : Constant  Value=0
  Create 3x3 Matrix : sharedutil/Create 3x3 Matrix  aMode=aMode
  Demux : Demux  Outputs=3
      settings: DisplayOption=none
  Gain : Gain  Gain=-1  SaturateOnIntegerOverflow=on  OutDataTypeStr=Inherit: Same as input  ParamDataTypeStr=Inherit: Same as input
  Gain1 : Gain  Gain=-1  SaturateOnIntegerOverflow=on  OutDataTypeStr=Inherit: Same as input  ParamDataTypeStr=Inherit: Same as input
  Gain2 : Gain  Gain=-1  SaturateOnIntegerOverflow=on  OutDataTypeStr=Inherit: Same as input  ParamDataTypeStr=Inherit: Same as input
  S(V) : Outport  VectorParamsAs1DForOutWhenUnconnected=off
  wires:
  Constant/1 -> Create 3x3 Matrix/1, Create 3x3 Matrix/9, Create 3x3 Matrix/5
  Demux/1 -> Gain/1, Create 3x3 Matrix/8  "v(1)"
  Demux/2 -> Gain1/1, Create 3x3 Matrix/3  "v(2)"
  Demux/3 -> Gain2/1, Create 3x3 Matrix/4  "v(3)"
  Gain/1 -> Create 3x3 Matrix/6  "-v(1)"
  Gain1/1 -> Create 3x3 Matrix/7  "-v(2)"
  Gain2/1 -> Create 3x3 Matrix/2  "-v(3)"
  Create 3x3 Matrix/1 -> S(V)/1
  v/1 -> Demux/1

== system RoboticFish_NGC/Robotic-Fish Model & PropulsionSystem/RF Dynamics and Kinematics (Attitude rappresentation: Quaternions)/6 DOF transformation/E2(e)/Skew Symmetrical Operator ==
  v : Inport
  Constant : Constant  Value=0
  Create 3x3 Matrix : sharedutil/Create 3x3 Matrix  aMode=aMode
  Demux : Demux  Outputs=3
      settings: DisplayOption=none
  Gain : Gain  Gain=-1  SaturateOnIntegerOverflow=on  OutDataTypeStr=Inherit: Same as input  ParamDataTypeStr=Inherit: Same as input
  Gain1 : Gain  Gain=-1  SaturateOnIntegerOverflow=on  OutDataTypeStr=Inherit: Same as input  ParamDataTypeStr=Inherit: Same as input
  Gain2 : Gain  Gain=-1  SaturateOnIntegerOverflow=on  OutDataTypeStr=Inherit: Same as input  ParamDataTypeStr=Inherit: Same as input
  S(V) : Outport  VectorParamsAs1DForOutWhenUnconnected=off
  wires:
  v/1 -> Demux/1
  Create 3x3 Matrix/1 -> S(V)/1
  Gain2/1 -> Create 3x3 Matrix/2  "-v(3)"
  Gain1/1 -> Create 3x3 Matrix/7  "-v(2)"
  Gain/1 -> Create 3x3 Matrix/6  "-v(1)"
  Demux/3 -> Create 3x3 Matrix/4, Gain2/1  "v(3)"
  Demux/2 -> Create 3x3 Matrix/3, Gain1/1  "v(2)"
  Demux/1 -> Create 3x3 Matrix/8, Gain/1  "v(1)"
  Constant/1 -> Create 3x3 Matrix/5, Create 3x3 Matrix/9, Create 3x3 Matrix/1

== system RoboticFish_NGC/Robotic-Fish Model & PropulsionSystem/RF Dynamics and Kinematics (Attitude rappresentation: Quaternions)/Restoring forces/E1(e)/Skew Symmetrical Operator ==
  v : Inport
  Constant : Constant  Value=0
  Create 3x3 Matrix : sharedutil/Create 3x3 Matrix  aMode=aMode
  Demux : Demux  Outputs=3
      settings: DisplayOption=none
  Gain : Gain  Gain=-1  SaturateOnIntegerOverflow=on  OutDataTypeStr=Inherit: Same as input  ParamDataTypeStr=Inherit: Same as input
  Gain1 : Gain  Gain=-1  SaturateOnIntegerOverflow=on  OutDataTypeStr=Inherit: Same as input  ParamDataTypeStr=Inherit: Same as input
  Gain2 : Gain  Gain=-1  SaturateOnIntegerOverflow=on  OutDataTypeStr=Inherit: Same as input  ParamDataTypeStr=Inherit: Same as input
  S(V) : Outport  VectorParamsAs1DForOutWhenUnconnected=off
  wires:
  v/1 -> Demux/1
  Create 3x3 Matrix/1 -> S(V)/1
  Gain2/1 -> Create 3x3 Matrix/2  "-v(3)"
  Gain1/1 -> Create 3x3 Matrix/7  "-v(2)"
  Gain/1 -> Create 3x3 Matrix/6  "-v(1)"
  Demux/3 -> Create 3x3 Matrix/4, Gain2/1  "v(3)"
  Demux/2 -> Create 3x3 Matrix/3, Gain1/1  "v(2)"
  Demux/1 -> Create 3x3 Matrix/8, Gain/1  "v(1)"
  Constant/1 -> Create 3x3 Matrix/5, Create 3x3 Matrix/9, Create 3x3 Matrix/1
